simulink model "Single_junction_MonteCarlo"  (R2019a)
settings: Solver=FixedStepAuto  StartTime=0.0  StopTime=1  FixedStep=dt  RelTol=1e-3
values from neighbouring files (symbols this model uses):
  phase_1 = 0    [initMonteCarlo.m]    (also in initTrapModel.m)
  phase_2 = 0.005    [initMonteCarlo.m]    (also in initTrapModel.m)
  Q1 = 0.5*60*1000000000    (= 30000000000)    [initMonteCarlo.m]    (also in initRealModel.m = 2000; initTrapModel.m)
  Q2 = 0.5*60*1000000000    (= 30000000000)    [initMonteCarlo.m]    (also in initRealModel.m = 2000; initTrapModel.m)
  rate_1 = 0.01    [initMonteCarlo.m]    (also in initTrapModel.m)
  rate_2 = 0.01    [initMonteCarlo.m]    (also in initTrapModel.m)
  seed_1 = 0    [initMonteCarlo.m]    (also in initRealModel.m; initTrapModel.m)
  seed_2 = 1    [initMonteCarlo.m]    (also in initRealModel.m; initTrapModel.m)
libraries: SinglePipe_lib x3, simulink x2, Junction_Lib x1
settings Model: Creator=martin  LastModifiedBy=martin

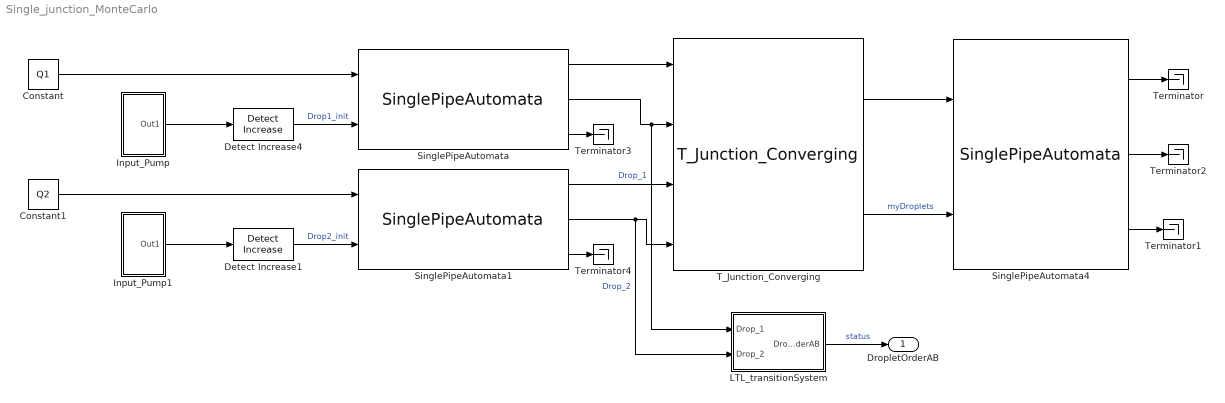
== system Single_junction_MonteCarlo ==
  Constant : Constant  Value=Q1
  Constant1 : Constant  Value=Q2
  Detect Increase1 : simulink/Logic and Bit Operations/Detect Increase  vinit=0  OutDataTypeStr=boolean
  Detect Increase4 : simulink/Logic and Bit Operations/Detect Increase  vinit=0  OutDataTypeStr=boolean
  Input_Pump : Subsystem  mask{Period=rate_1, Seed=seed_1, PhaseDelay=phase_1}
      mask prompts: Period "droplet rate"; Seed "Simulink:blkprm_prompts:RandNumInitSeed"; PhaseDelay "Simulink:blkprm_prompts:PulseContPhaseDelay"
      mask TypeOptions Period:
      | Pulse
      | Generator/Period
      mask TypeOptions Seed:
      | Uniform Random
      | Number4/Seed
      mask TypeOptions PhaseDelay:
      | Pulse
      | Generator/PhaseDelay
      mask DialogControl Seed Prompt: Seed:
      mask DialogControl PhaseDelay Prompt: Phase delay (secs):
  Input_Pump1 : Subsystem  mask{Period=rate_2, Seed=seed_2, PhaseDelay=phase_2}
      mask prompts: Period "droplet rate"; Seed "Simulink:blkprm_prompts:RandNumInitSeed"; PhaseDelay "Simulink:blkprm_prompts:PulseContPhaseDelay"
      mask TypeOptions Period:
      | Pulse
      | Generator/Period
      mask TypeOptions Seed:
      | Uniform Random
      | Number4/Seed
      mask TypeOptions PhaseDelay:
      | Pulse
      | Generator/PhaseDelay
      mask DialogControl Seed Prompt: Seed:
      mask DialogControl PhaseDelay Prompt: Phase delay (secs):
  LTL_transitionSystem : Subsystem
  SinglePipeAutomata : SinglePipe_lib/SinglePipeAutomata  width=W_A  length=L_A  height=H_A  dt=dt
  SinglePipeAutomata1 : SinglePipe_lib/SinglePipeAutomata  width=W_B  length=L_B  height=H_B  dt=dt
  SinglePipeAutomata4 : SinglePipe_lib/SinglePipeAutomata  width=W_C  length=L_C  height=H_C  dt=dt
  T_Junction_Converging : Junction_Lib/T_Junction_Converging  SystemSampleTime=-1
  Terminator{,1..4} (5 alike) : Terminator
  DropletOrderAB : Outport
  wires:
  Detect Increase1/1 -> SinglePipeAutomata1/2  "Drop2_init"
  Input_Pump/1(Out1) -> Detect Increase4/1
  SinglePipeAutomata/1 -> T_Junction_Converging/1
  SinglePipeAutomata1/3 -> Terminator4/1
  SinglePipeAutomata4/3 -> Terminator1/1
  SinglePipeAutomata1/2 -> LTL_transitionSystem/2(Drop_2), T_Junction_Converging/4  "Drop_2"
  Input_Pump1/1(Out1) -> Detect Increase1/1
  Constant/1 -> SinglePipeAutomata/1
  SinglePipeAutomata/3 -> Terminator3/1
  SinglePipeAutomata/2 -> LTL_transitionSystem/1(Drop_1), T_Junction_Converging/2  "Drop_1"
  Constant1/1 -> SinglePipeAutomata1/1
  T_Junction_Converging/2 -> SinglePipeAutomata4/2  "myDroplets"
  T_Junction_Converging/1 -> SinglePipeAutomata4/1
  SinglePipeAutomata1/1 -> T_Junction_Converging/3
  Detect Increase4/1 -> SinglePipeAutomata/2  "Drop1_init"
  SinglePipeAutomata4/1 -> Terminator/1
  SinglePipeAutomata4/2 -> Terminator2/1
  LTL_transitionSystem/1(DropletOrderAB) -> DropletOrderAB/1  "status"

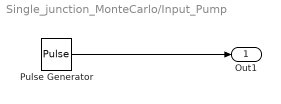
== system Single_junction_MonteCarlo/Input_Pump ==
  Pulse Generator : DiscretePulseGenerator  PulseType=Time based  Period=Period  PulseWidth=50  PhaseDelay=PhaseDelay
  Out1 : Outport
  wires:
  Pulse Generator/1 -> Out1/1

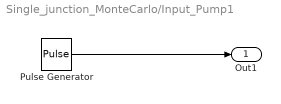
== system Single_junction_MonteCarlo/Input_Pump1 ==
  Pulse Generator : DiscretePulseGenerator  PulseType=Time based  Period=Period  PulseWidth=50  PhaseDelay=PhaseDelay
  Out1 : Outport
  wires:
  Pulse Generator/1 -> Out1/1

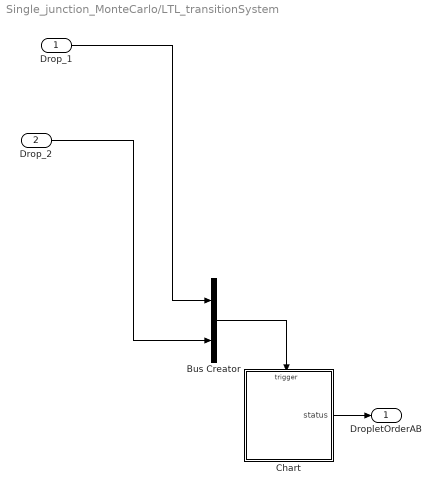
== system Single_junction_MonteCarlo/LTL_transitionSystem ==
  Drop_1 : Inport
  Drop_2 : Inport  Port=2
  Bus Creator : BusCreator  Inputs=2
  Chart : Stateflow chart  BlockKeywords=__PRM__SERIALIZED__DATA__:Stateflow Chart,Stateflow Diagram  TreatAsAtomicUnit=on
  DropletOrderAB : Outport
  wires:
  Bus Creator/1 -> Chart/Trigger
  Chart/1(status) -> DropletOrderAB/1
  Drop_2/1 -> Bus Creator/2
  Drop_1/1 -> Bus Creator/1

== stateflow chart Single_junction_MonteCarlo/LTL_transitionSystem/Chart ==
  state null
    en:status=0;
  state State_A
    en:status=1;
  state Error
    en:status=2;
  state State_B
    en:status=1;
  (default) -> null [order 3]
  (default) -> State_A [order 1] : Drop_1
  null -> State_A [order 1] : Drop_1
  State_A -> State_B [order 1] : Drop_2
  Error -> State_A [order 1] : Drop_1
  State_A -> Error [order 2] : Drop_1
  State_B -> State_A [order 1] : Drop_1
  null -> State_B [order 2] : Drop_2
  (default) -> State_B [order 2] : Drop_2
  Error -> State_B [order 2] : Drop_2
  State_B -> Error [order 2] : Drop_2
  data: status output =-1
  events: Drop_1 input RISING_EDGE_EVENT; Drop_2 input RISING_EDGE_EVENT
